simulink model "test_ibob_data_mux_10_1"  (Simulink 7.0)
settings: Solver=ode45  StartTime=0.0  StopTime=3000  RelTol=1e-3
libraries: xbsIndex_r4 x218, xbsReplacements_r4 x24, xps_library x3, xbsIndex_r3 x1
(part 2 of 2)

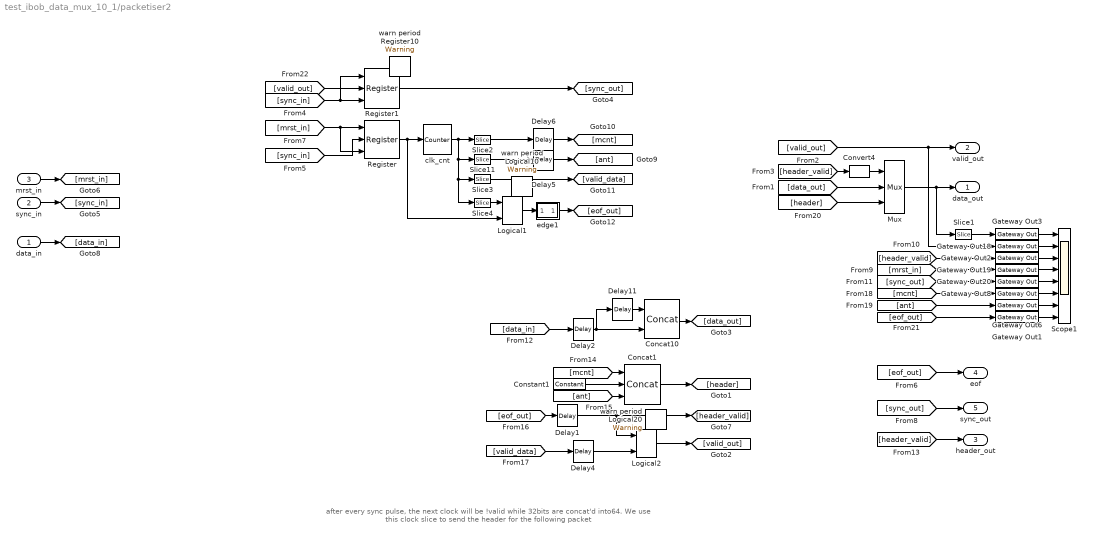
== system test_ibob_data_mux_10_1/packetiser2 ==
  note: after every sync pulse,
      | the next clock will be !valid while 32bits are concat'd into64.
      | We use this clock slice to send the header for the following packet
  data_in : Inport  OutDataType=sfix(16)  OutScaling=2^0
  sync_in : Inport  Port=2  OutDataType=sfix(16)  OutScaling=2^0
  mrst_in : Inport  Port=3  OutDataType=sfix(16)  OutScaling=2^0
  Concat1 : xbsIndex_r4/Concat  num_inputs=3  dbl_ovrd=off  block_type=concat
      settings: block_version=10.1.3
  Concat10 : xbsIndex_r4/Concat  num_inputs=2  dbl_ovrd=off  block_type=concat
      settings: block_version=10.1.3
  Constant1 : xbsIndex_r4/Constant  arith_type=Unsigned  const=0  n_bits=16-ant_bits  bin_pt=0  explicit_period=on  period=1  equ=P=C  opselect=C  inp2=PCIN>>17  opr=+  inp1=P  carry=CIN  dbl_ovrd=off  block_type=constant
  Convert4 : xbsIndex_r4/Convert  arith_type=Unsigned  n_bits=1  bin_pt=0  quantization=Truncate  overflow=Wrap  latency=0  dbl_ovrd=off  pipeline=off  block_type=convert
      settings: xl_area=[0, 0, 0, 0, 0, 0, 0]  block_version=10.1.3
  Delay{1..2,4..6,11} (6 alike) : xbsIndex_r4/Delay  en=off  latency=1  dbl_ovrd=off  reg_retiming=on  block_type=delay
      settings: xl_area=[0, 0, 0, 0, 0, 0, 0]
  Gateway Out{1..3,6,8,18..20} (8 alike) : xbsIndex_r4/Gateway Out  hdl_port=on  timing_constraint=None  locs_specified=off  LOCs={}  block_type=gatewayout
      settings: infoedit="Gateway out block.  Converts Xilinx fixed point inputs into ouputs of type Simulink integer, double, or fixed point.<P><P>Hardware notes:  In hardware these blocks become top level output ports or are discarded, depending on how they are configured."  xl_area=[0, 0, 0, 0, 0, 0, 0]  block_version=10.1.3
  Logical1 : xbsIndex_r4/Logical  logical_function=OR  inputs=2  en=off  latency=0  precision=Full  arith_type=Unsigned  n_bits=1  bin_pt=0  align_bp=on  dbl_ovrd=off  block_type=logical
      settings: xl_area=[0, 0, 0, 0, 0, 0, 0]
  Logical2 : xbsIndex_r4/Logical  logical_function=OR  inputs=2  en=off  latency=0  precision=Full  arith_type=Unsigned  n_bits=1  bin_pt=0  align_bp=on  dbl_ovrd=off  block_type=logical
      settings: xl_area=[0, 0, 0, 0, 0, 0, 0]
  Mux : xbsIndex_r4/Mux  inputs=2  en=off  latency=0  precision=Full  arith_type="Signed  (2's comp)"  n_bits=8  bin_pt=2  quantization=Truncate  overflow=Wrap  dbl_ovrd=off  block_type=mux
      settings: xl_area=[0, 0, 0, 0, 0, 0, 0]
  Register : xbsIndex_r4/Register  init=0  rst=on  en=on  dbl_ovrd=off  block_type=register
      settings: xl_area=[0, 0, 0, 0, 0, 0, 0]
  Register1 : xbsIndex_r4/Register  init=0  rst=on  en=on  dbl_ovrd=off  block_type=register
      settings: xl_area=[0, 0, 0, 0, 0, 0, 0]
  Scope1 : Scope  NumInputPorts=8
      settings: YMin=0~0~0~-1~-1~-5~-5~-5  YMax=4e+013~1~1~1~1~5~5~5  SaveName=ScopeData6
  Slice1 : xbsIndex_r4/Slice  nbits=32  boolean_output=off  mode=Lower Bit Location + Width  bit1=0  base1=MSB of Input  bit0=0  base0=LSB of Input  dbl_ovrd=off  block_type=slice
      settings: infoedit="Extracts a given range of bits from each input sample and presents it at the output.  The output type is ordinarily unsigned with binary point at zero, but can be Boolean when the slice is one bit wide.<P><P>Hardware notes: In hardware this block costs nothing."  block_version=10.1.3
  Slice11 : xbsIndex_r4/Slice  nbits=ant_bits  boolean_output=on  mode=Lower Bit Location + Width  bit1=0  base1=MSB of Input  bit0=nwrd_bits+1  base0=LSB of Input  dbl_ovrd=off  block_type=slice
      settings: infoedit="Extracts a given range of bits from each input sample and presents it at the output.  The output type is ordinarily unsigned with binary point at zero, but can be Boolean when the slice is one bit wide.<P><P>Hardware notes: In hardware this block costs nothing."  block_version=10.1.3
  Slice2 : xbsIndex_r4/Slice  nbits=48  boolean_output=off  mode=Upper Bit Location + Width  bit1=0  base1=MSB of Input  bit0=0  base0=LSB of Input  dbl_ovrd=off  block_type=slice
      settings: infoedit="Extracts a given range of bits from each input sample and presents it at the output.  The output type is ordinarily unsigned with binary point at zero, but can be Boolean when the slice is one bit wide.<P><P>Hardware notes: In hardware this block costs nothing."  block_version=10.1.3
  Slice3 : xbsIndex_r4/Slice  nbits=1  boolean_output=on  mode=Lower Bit Location + Width  bit1=0  base1=MSB of Input  bit0=0  base0=LSB of Input  dbl_ovrd=off  block_type=slice
      settings: infoedit="Extracts a given range of bits from each input sample and presents it at the output.  The output type is ordinarily unsigned with binary point at zero, but can be Boolean when the slice is one bit wide.<P><P>Hardware notes: In hardware this block costs nothing."  block_version=10.1.3
  Slice4 : xbsIndex_r4/Slice  nbits=1  boolean_output=on  mode=Lower Bit Location + Width  bit1=0  base1=MSB of Input  bit0=nwrd_bits+1  base0=LSB of Input  dbl_ovrd=off  block_type=slice
      settings: infoedit="Extracts a given range of bits from each input sample and presents it at the output.  The output type is ordinarily unsigned with binary point at zero, but can be Boolean when the slice is one bit wide.<P><P>Hardware notes: In hardware this block costs nothing."  block_version=10.1.3
  clk_cnt : xbsIndex_r4/Counter  cnt_type=Free Running  cnt_to=Inf  operation=Up  start_count=0  cnt_by_val=1  arith_type=Unsigned  n_bits=48+nwrd_bits+ant_bits+1  bin_pt=0  load_pin=off  rst=on  en=off  explicit_period=off  period=1  dbl_ovrd=off  use_behavioral_HDL=off  use_rpm=on  implementation=Fabric  block_type=counter
      settings: xl_area=[0, 0, 0, 0, 0, 0, 0]
  edge1 : Subsystem
      mask Type: edge
      mask Description: Outputs true if a boolean input signal is not equal to its value last clock.
      mask Help: eval('xlWeb([getenv(''MLIB_ROOT''), ''\casper_library\doc\edge_usage.html''])')
  warn period Logical10 : xbsReplacements_r4/Warning  SystemSampleTime=-1  period=1
  warn period Logical20 : xbsReplacements_r4/Warning  SystemSampleTime=-1  period=1
  warn period Register10 : xbsReplacements_r4/Warning  SystemSampleTime=-1  period=1
  data_out : Outport  OutDataType=sfix(16)  OutScaling=2^0
  valid_out : Outport  Port=2  OutDataType=sfix(16)  OutScaling=2^0
  header_out : Outport  Port=3  OutDataType=sfix(16)  OutScaling=2^0
  eof : Outport  Port=4  OutDataType=sfix(16)  OutScaling=2^0
  sync_out : Outport  Port=5  OutDataType=sfix(16)  OutScaling=2^0
  wires:
  Constant1/1 -> Concat1/2
  Convert4/1 -> Mux/1
  Mux/1 -> data_out/1, Slice1/1
  Concat1/1 -> [header]
  [header] -> Mux/3
  [data_out] -> Mux/2
  [valid_out] -> valid_out/1, Gateway Out18/1
  [header_valid] -> Convert4/1
  sync_in/1 -> [sync_in]
  mrst_in/1 -> [mrst_in]
  Register/1 -> Logical1/2, clk_cnt/1
  [eof_out] -> eof/1
  [sync_out] -> sync_out/1
  Gateway Out3/1 -> Scope1/1
  Gateway Out18/1 -> Scope1/2
  Gateway Out2/1 -> Scope1/3
  Gateway Out19/1 -> Scope1/4
  Gateway Out20/1 -> Scope1/5
  [header_valid] -> Gateway Out2/1
  [mrst_in] -> Gateway Out19/1
  [sync_out] -> Gateway Out20/1
  [sync_in] -> Register1/3, Register1/1
  [eof_out] -> Delay1/1
  Concat10/1 -> [data_out]
  [mrst_in] -> Register/1, Register/3
  [sync_in] -> Register/2
  [header_valid] -> header_out/1
  Logical2/1 -> [valid_out]
  clk_cnt/1 -> Slice2/1, Slice11/1, Slice3/1, Slice4/1
  [mcnt] -> Concat1/1
  [ant] -> Concat1/3
  Slice2/1 -> Delay6/1
  Slice11/1 -> Delay5/1
  Slice3/1 -> [valid_data]
  Slice4/1 -> Logical1/1
  [valid_data] -> Delay4/1
  Gateway Out8/1 -> Scope1/6
  [mcnt] -> Gateway Out8/1
  Logical1/1 -> edge1/1(in)
  edge1/1(out) -> [eof_out]
  Gateway Out6/1 -> Scope1/7
  [ant] -> Gateway Out6/1
  [data_in] -> Delay2/1
  Delay11/1 -> Concat10/1
  data_in/1 -> [data_in]
  Slice1/1 -> Gateway Out3/1
  Gateway Out1/1 -> Scope1/8
  [eof_out] -> Gateway Out1/1
  Register1/1 -> [sync_out]
  Delay1/1 -> Logical2/1, [header_valid]
  Delay2/1 -> Concat10/2, Delay11/1
  Delay4/1 -> Logical2/2
  Delay5/1 -> [ant]
  Delay6/1 -> [mcnt]
  [valid_out] -> Register1/2

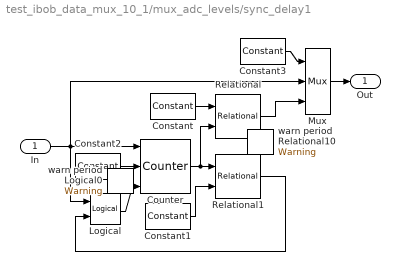
== system test_ibob_data_mux_10_1/mux_adc_levels/sync_delay1 ==
  In : Inport  OutDataType=sfix(16)  OutScaling=2^0
  Constant : xbsIndex_r4/Constant  arith_type=Unsigned  const=1  n_bits=BitWidth  bin_pt=0  explicit_period=on  period=1  equ=P=C  opselect=C  inp2=PCIN>>17  opr=+  inp1=P  carry=CIN  dbl_ovrd=off  block_type=constant
  Constant1 : xbsIndex_r4/Constant  arith_type=Unsigned  const=0  n_bits=BitWidth  bin_pt=0  explicit_period=on  period=1  equ=P=C  opselect=C  inp2=PCIN>>17  opr=+  inp1=P  carry=CIN  dbl_ovrd=off  block_type=constant
  Constant2 : xbsIndex_r4/Constant  arith_type=Unsigned  const=DelayLen  n_bits=BitWidth  bin_pt=0  explicit_period=on  period=1  equ=P=C  opselect=C  inp2=PCIN>>17  opr=+  inp1=P  carry=CIN  dbl_ovrd=off  block_type=constant
  Constant3 : xbsIndex_r4/Constant  arith_type=Unsigned  const=UseCounter  n_bits=1  bin_pt=0  explicit_period=on  period=1  equ=P=C  opselect=C  inp2=PCIN>>17  opr=+  inp1=P  carry=CIN  dbl_ovrd=off  block_type=constant
  Counter : xbsIndex_r4/Counter  cnt_type=Free Running  cnt_to=Inf  operation=Down  start_count=0  cnt_by_val=1  arith_type=Unsigned  n_bits=BitWidth  bin_pt=0  load_pin=on  rst=off  en=on  explicit_period=on  period=1  dbl_ovrd=off  use_behavioral_HDL=off  use_rpm=on  implementation=Fabric  block_type=counter
      settings: xl_area=[0, 0, 0, 0, 0, 0, 0]
  Logical : xbsIndex_r4/Logical  logical_function=OR  inputs=2  en=off  latency=0  precision=Full  arith_type=Unsigned  n_bits=8  bin_pt=2  align_bp=on  dbl_ovrd=off  block_type=logical
      settings: xl_area=[0, 0, 0, 0, 0, 0, 0]
  Mux : xbsIndex_r4/Mux  inputs=2  en=off  latency=0  precision=Full  arith_type="Signed  (2's comp)"  n_bits=8  bin_pt=2  quantization=Truncate  overflow=Wrap  dbl_ovrd=off  block_type=mux
      settings: xl_area=[0, 0, 0, 0, 0, 0, 0]
  Relational : xbsIndex_r4/Relational  mode=a=b  en=off  latency=0  dbl_ovrd=off  block_type=relational
      settings: xl_area=[0, 0, 0, 0, 0, 0, 0]  block_version=10.1.3
  Relational1 : xbsIndex_r4/Relational  mode=a!=b  en=off  latency=0  dbl_ovrd=off  block_type=relational
      settings: xl_area=[0, 0, 0, 0, 0, 0, 0]  block_version=10.1.3
  warn period Logical0 : xbsReplacements_r4/Warning  SystemSampleTime=-1  period=1
  warn period Relational10 : xbsReplacements_r4/Warning  SystemSampleTime=-1  period=1
  Out : Outport  OutDataType=sfix(16)  OutScaling=2^0
  wires:
  Counter/1 -> Relational1/1, Relational/2
  Constant1/1 -> Relational1/2
  Constant/1 -> Relational/1
  Constant2/1 -> Counter/2
  In/1 -> Counter/1, Logical/1, Mux/2
  Logical/1 -> Counter/3
  Relational1/1 -> Logical/2
  Relational/1 -> Mux/3
  Constant3/1 -> Mux/1
  Mux/1 -> Out/1

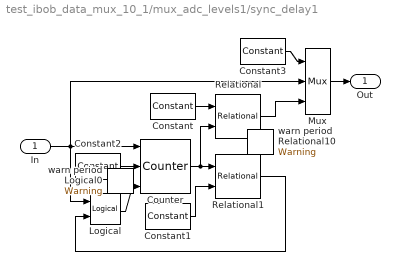
== system test_ibob_data_mux_10_1/mux_adc_levels1/sync_delay1 ==
  In : Inport  OutDataType=sfix(16)  OutScaling=2^0
  Constant : xbsIndex_r4/Constant  arith_type=Unsigned  const=1  n_bits=BitWidth  bin_pt=0  explicit_period=on  period=1  equ=P=C  opselect=C  inp2=PCIN>>17  opr=+  inp1=P  carry=CIN  dbl_ovrd=off  block_type=constant
  Constant1 : xbsIndex_r4/Constant  arith_type=Unsigned  const=0  n_bits=BitWidth  bin_pt=0  explicit_period=on  period=1  equ=P=C  opselect=C  inp2=PCIN>>17  opr=+  inp1=P  carry=CIN  dbl_ovrd=off  block_type=constant
  Constant2 : xbsIndex_r4/Constant  arith_type=Unsigned  const=DelayLen  n_bits=BitWidth  bin_pt=0  explicit_period=on  period=1  equ=P=C  opselect=C  inp2=PCIN>>17  opr=+  inp1=P  carry=CIN  dbl_ovrd=off  block_type=constant
  Constant3 : xbsIndex_r4/Constant  arith_type=Unsigned  const=UseCounter  n_bits=1  bin_pt=0  explicit_period=on  period=1  equ=P=C  opselect=C  inp2=PCIN>>17  opr=+  inp1=P  carry=CIN  dbl_ovrd=off  block_type=constant
  Counter : xbsIndex_r4/Counter  cnt_type=Free Running  cnt_to=Inf  operation=Down  start_count=0  cnt_by_val=1  arith_type=Unsigned  n_bits=BitWidth  bin_pt=0  load_pin=on  rst=off  en=on  explicit_period=on  period=1  dbl_ovrd=off  use_behavioral_HDL=off  use_rpm=on  implementation=Fabric  block_type=counter
      settings: xl_area=[0, 0, 0, 0, 0, 0, 0]
  Logical : xbsIndex_r4/Logical  logical_function=OR  inputs=2  en=off  latency=0  precision=Full  arith_type=Unsigned  n_bits=8  bin_pt=2  align_bp=on  dbl_ovrd=off  block_type=logical
      settings: xl_area=[0, 0, 0, 0, 0, 0, 0]
  Mux : xbsIndex_r4/Mux  inputs=2  en=off  latency=0  precision=Full  arith_type="Signed  (2's comp)"  n_bits=8  bin_pt=2  quantization=Truncate  overflow=Wrap  dbl_ovrd=off  block_type=mux
      settings: xl_area=[0, 0, 0, 0, 0, 0, 0]
  Relational : xbsIndex_r4/Relational  mode=a=b  en=off  latency=0  dbl_ovrd=off  block_type=relational
      settings: xl_area=[0, 0, 0, 0, 0, 0, 0]  block_version=10.1.3
  Relational1 : xbsIndex_r4/Relational  mode=a!=b  en=off  latency=0  dbl_ovrd=off  block_type=relational
      settings: xl_area=[0, 0, 0, 0, 0, 0, 0]  block_version=10.1.3
  warn period Logical0 : xbsReplacements_r4/Warning  SystemSampleTime=-1  period=1
  warn period Relational10 : xbsReplacements_r4/Warning  SystemSampleTime=-1  period=1
  Out : Outport  OutDataType=sfix(16)  OutScaling=2^0
  wires:
  Counter/1 -> Relational1/1, Relational/2
  Constant1/1 -> Relational1/2
  Constant/1 -> Relational/1
  Constant2/1 -> Counter/2
  In/1 -> Counter/1, Logical/1, Mux/2
  Logical/1 -> Counter/3
  Relational1/1 -> Logical/2
  Relational/1 -> Mux/3
  Constant3/1 -> Mux/1
  Mux/1 -> Out/1

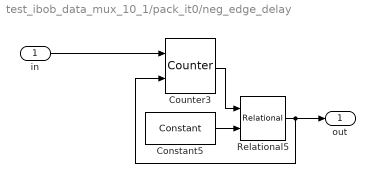
== system test_ibob_data_mux_10_1/pack_it0/neg_edge_delay ==
  in : Inport  OutDataType=sfix(16)  OutScaling=2^0
  Constant5 : xbsIndex_r4/Constant  arith_type=Unsigned  const=pulse_len  n_bits=bits  bin_pt=0  explicit_period=off  period=1  equ=P=C  opselect=C  inp2=PCIN>>17  opr=+  inp1=P  carry=CIN  dbl_ovrd=off  block_type=constant
  Counter3 : xbsIndex_r4/Counter  cnt_type=Free Running  cnt_to=1023  operation=Up  start_count=0  cnt_by_val=1  arith_type=Unsigned  n_bits=bits  bin_pt=0  load_pin=off  rst=on  en=on  explicit_period=on  period=1  dbl_ovrd=off  use_behavioral_HDL=off  use_rpm=on  implementation=Fabric  block_type=counter
      settings: xl_area=[0, 0, 0, 0, 0, 0, 0]
  Relational5 : xbsIndex_r4/Relational  mode=a!=b  en=off  latency=0  dbl_ovrd=off  block_type=relational
      settings: xl_area=[0, 0, 0, 0, 0, 0, 0]  block_version=10.1.3
  out : Outport  OutDataType=sfix(16)  OutScaling=2^0
  wires:
  Relational5/1 -> out/1, Counter3/2
  Constant5/1 -> Relational5/2
  Counter3/1 -> Relational5/1
  in/1 -> Counter3/1

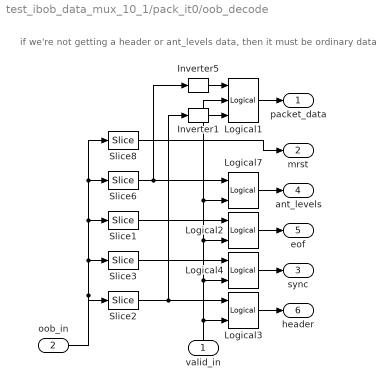
== system test_ibob_data_mux_10_1/pack_it0/oob_decode ==
  note: if we're not getting a header or ant_levels data,
      | then it must be ordinary data
  valid_in : Inport  Orientation=up  OutDataType=sfix(16)  OutScaling=2^0
  oob_in : Inport  Port=2  OutDataType=sfix(16)  OutScaling=2^0
  Inverter1 : xbsIndex_r4/Inverter  en=off  latency=0  dbl_ovrd=off  block_type=inv
      settings: xl_area=[0, 0, 0, 0, 0, 0, 0]
  Inverter5 : xbsIndex_r4/Inverter  en=off  latency=0  dbl_ovrd=off  block_type=inv
      settings: xl_area=[0, 0, 0, 0, 0, 0, 0]
  Logical1 : xbsIndex_r4/Logical  logical_function=AND  inputs=3  en=off  latency=0  precision=Full  arith_type=Unsigned  n_bits=8  bin_pt=2  align_bp=on  dbl_ovrd=off  block_type=logical
      settings: xl_area=[0, 0, 0, 0, 0, 0, 0]
  Logical{2..4,7} (4 alike) : xbsIndex_r4/Logical  logical_function=AND  inputs=2  en=off  latency=0  precision=Full  arith_type=Unsigned  n_bits=8  bin_pt=2  align_bp=on  dbl_ovrd=off  block_type=logical
      settings: xl_area=[0, 0, 0, 0, 0, 0, 0]
  Slice1 : xbsIndex_r4/Slice  nbits=1  boolean_output=on  mode=Lower Bit Location + Width  bit1=0  base1=MSB of Input  bit0=2  base0=LSB of Input  dbl_ovrd=off  block_type=slice
      settings: infoedit="Extracts a given range of bits from each input sample and presents it at the output.  The output type is ordinarily unsigned with binary point at zero, but can be Boolean when the slice is one bit wide.<P><P>Hardware notes: In hardware this block costs nothing."  block_version=10.1.3
  Slice2 : xbsIndex_r4/Slice  nbits=1  boolean_output=on  mode=Lower Bit Location + Width  bit1=0  base1=MSB of Input  bit0=0  base0=LSB of Input  dbl_ovrd=off  block_type=slice
      settings: infoedit="Extracts a given range of bits from each input sample and presents it at the output.  The output type is ordinarily unsigned with binary point at zero, but can be Boolean when the slice is one bit wide.<P><P>Hardware notes: In hardware this block costs nothing."  block_version=10.1.3
  Slice3 : xbsIndex_r4/Slice  nbits=1  boolean_output=on  mode=Lower Bit Location + Width  bit1=0  base1=MSB of Input  bit0=1  base0=LSB of Input  dbl_ovrd=off  block_type=slice
      settings: infoedit="Extracts a given range of bits from each input sample and presents it at the output.  The output type is ordinarily unsigned with binary point at zero, but can be Boolean when the slice is one bit wide.<P><P>Hardware notes: In hardware this block costs nothing."  block_version=10.1.3
  Slice6 : xbsIndex_r4/Slice  nbits=1  boolean_output=on  mode=Lower Bit Location + Width  bit1=0  base1=MSB of Input  bit0=3  base0=LSB of Input  dbl_ovrd=off  block_type=slice
      settings: infoedit="Extracts a given range of bits from each input sample and presents it at the output.  The output type is ordinarily unsigned with binary point at zero, but can be Boolean when the slice is one bit wide.<P><P>Hardware notes: In hardware this block costs nothing."  block_version=10.1.3
  Slice8 : xbsIndex_r4/Slice  nbits=1  boolean_output=on  mode=Lower Bit Location + Width  bit1=0  base1=MSB of Input  bit0=4  base0=LSB of Input  dbl_ovrd=off  block_type=slice
      settings: infoedit="Extracts a given range of bits from each input sample and presents it at the output.  The output type is ordinarily unsigned with binary point at zero, but can be Boolean when the slice is one bit wide.<P><P>Hardware notes: In hardware this block costs nothing."  block_version=10.1.3
  packet_data : Outport  OutDataType=sfix(16)  OutScaling=2^0
  mrst : Outport  Port=2  OutDataType=sfix(16)  OutScaling=2^0
  sync : Outport  Port=3  OutDataType=sfix(16)  OutScaling=2^0
  ant_levels : Outport  Port=4  OutDataType=sfix(16)  OutScaling=2^0
  eof : Outport  Port=5  OutDataType=sfix(16)  OutScaling=2^0
  header : Outport  Port=6  OutDataType=sfix(16)  OutScaling=2^0
  wires:
  Slice8/1 -> mrst/1
  oob_in/1 -> Slice3/1, Slice1/1, Slice6/1, Slice8/1, Slice2/1
  valid_in/1 -> Logical3/2, Logical2/2, Logical7/2, Logical1/2, Logical4/2
  Logical1/1 -> packet_data/1
  Inverter5/1 -> Logical1/1
  Logical7/1 -> ant_levels/1
  Slice1/1 -> Logical2/1
  Logical2/1 -> eof/1
  Slice6/1 -> Logical7/1, Inverter5/1
  Slice2/1 -> Logical3/1, Inverter1/1
  Logical3/1 -> header/1
  Inverter1/1 -> Logical1/3
  Slice3/1 -> Logical4/1
  Logical4/1 -> sync/1

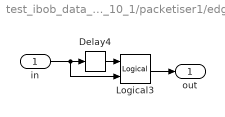
== system test_ibob_data_mux_10_1/packetiser1/edge ==
  in : Inport  OutDataType=sfix(16)  OutScaling=2^0
  Delay4 : xbsIndex_r4/Delay  en=off  latency=1  dbl_ovrd=off  reg_retiming=off  block_type=delay
      settings: xl_area=[0, 0, 0, 0, 0, 0, 0]
  Logical3 : xbsIndex_r4/Logical  logical_function=XOR  inputs=2  en=off  latency=0  precision=Full  arith_type=Unsigned  n_bits=8  bin_pt=2  align_bp=on  dbl_ovrd=off  block_type=logical
      settings: xl_area=[0, 0, 0, 0, 0, 0, 0]
  out : Outport  OutDataType=sfix(16)  OutScaling=2^0
  wires:
  in/1 -> Logical3/2, Delay4/1
  Delay4/1 -> Logical3/1
  Logical3/1 -> out/1

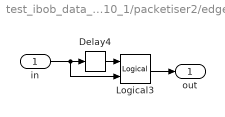
== system test_ibob_data_mux_10_1/packetiser2/edge1 ==
  in : Inport  OutDataType=sfix(16)  OutScaling=2^0
  Delay4 : xbsIndex_r4/Delay  en=off  latency=1  dbl_ovrd=off  reg_retiming=off  block_type=delay
      settings: xl_area=[0, 0, 0, 0, 0, 0, 0]
  Logical3 : xbsIndex_r4/Logical  logical_function=XOR  inputs=2  en=off  latency=0  precision=Full  arith_type=Unsigned  n_bits=8  bin_pt=2  align_bp=on  dbl_ovrd=off  block_type=logical
      settings: xl_area=[0, 0, 0, 0, 0, 0, 0]
  out : Outport  OutDataType=sfix(16)  OutScaling=2^0
  wires:
  Logical3/1 -> out/1
  Delay4/1 -> Logical3/1
  in/1 -> Delay4/1, Logical3/2
